simulink model "rtwdemo_cppencap"  (Simulink 7.6)
settings: Solver=FixedStepDiscrete  SolverMode=SingleTasking  StartTime=0.0  StopTime=100.0  FixedStep=0.1  RelTol=1e-3
PostLoadFcn:
  | rtwdemo_cppencap_data
libraries: rtwdemowidgets x1
Description:
  | C++ Classes for Models
settings Model: Creator=The MathWorks Inc.  CovMetricSettings=d  ExtModeAutoUpdateStatusClock=off
settings DataIOCC: SaveOutput=off  SaveTime=off  SignalLoggingName=sigsOut
settings OptimizationCC: InlineParams=on  InlineInvariantSignals=on  PassReuseOutputArgsAs=Individual arguments  StateBitsets=on  DataBitsets=on  UseTempVars=on  ZeroExternalMemoryAtStartup=off  ZeroInternalMemoryAtStartup=off  NoFixptDivByZeroProtection=on  EfficientFloat2IntCast=on  OptimizeModelRefInitCode=on  LifeSpan=1
settings DebuggingCC: SignalInfNanChecking=error  AlgebraicLoopMsg=error  ArtificialAlgebraicLoopMsg=error  UnderspecifiedInitializationDetection=Simplified  MergeDetectMultiDrivingBlocksExec=error  CheckExecutionContextPreStartOutputMsg=on  CheckExecutionContextRuntimeOutputMsg=on  BlockPriorityViolationMsg=error  MinStepSizeMsg=error  SolverPrmCheckMsg=error  InheritedTsInSrcMsg=error  DiscreteInheritContinuousMsg=error  SingleTaskRateTransMsg=error  TasksWithSamePriorityMsg=error  SigSpecEnsureSampleTimeMsg=error  CheckMatrixSingularityMsg=error  IntegerOverflowMsg=error  ParameterUnderflowMsg=error  ParameterPrecisionLossMsg=error  ParameterTunabilityLossMsg=error  UnderSpecifiedDataTypeMsg=error  UniqueDataStoreMsg=error  UnknownTsInhSupMsg=error  StrictBusMsg=ErrorOnBusTreatedAsVector
settings HardwareCC: ProdIntDivRoundTo=Zero  ProdEndianess=LittleEndian  ProdHWDeviceType=Generic->32-bit Embedded Processor  TargetHWDeviceType=Generic->32-bit Embedded Processor
settings SFSimCC: SimParseCustomCode=off
settings RTWCC: SystemTargetFile=ert.tlc  TLCOptions=-p0  TemplateMakefile=ert_default_tmf  Description=Real-Time Workshop Embedded Coder (no auto configuration)  GenerateReport=on  RTWVerbose=off  ProcessScript=ert_make_rtw_hook  IncludeHyperlinkInReport=on  LaunchReport=on  TargetLang=C++ (Encapsulated)  GenerateTraceInfo=on  GenerateTraceReport=on  GenerateTraceReportSl=on  GenerateTraceReportSf=on  GenerateTraceReportEml=on
settings CodeAppCC: ForceParamTrailComments=on  IgnoreTestpoints=on  MaxIdLength=128  SimulinkDataObjDesc=on  CustomSymbolStrGlobalVar=rt$N$M  CustomSymbolStrType=$N$M  CustomSymbolStrFcn=$N$M$F  CustomSymbolStrMacro=$N$M  InsertBlockDesc=on
settings ERTTargetCC: MultiwordLength=2048  GenerateSampleERTMain=on  IncludeMdlTerminateFcn=off  MultiInstanceERTCode=on  SupportNonFinite=off  SupportComplex=off  InlinedParameterPlacement=NonHierarchical  RootIOFormat=Structure reference  ERTCustomFileTemplate=example_file_process.tlc  ConvertIfToSwitch=off
settings ERTCPPComponent: GenerateDestructor=on  GenerateExternalIOAccessMethods=None  ParameterMemberVisibility=private  InternalMemberVisibility=private  GenerateParameterAccessMethods=None  GenerateInternalMemberAccessMethods=None  UseOperatorNewForModelRefRegistration=off

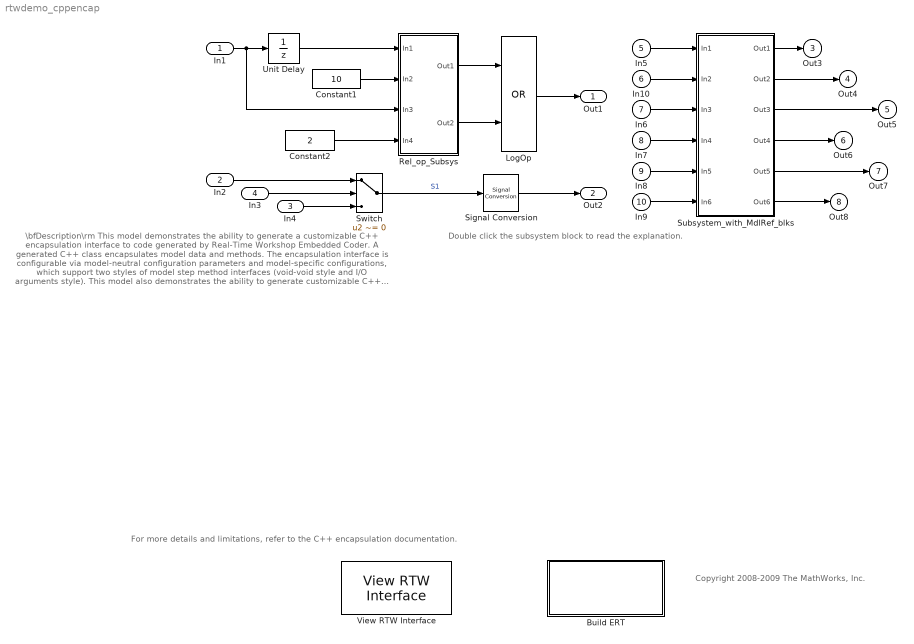
== system rtwdemo_cppencap ==
  note: \bfDescription\rm
      | This model demonstrates the ability to generate a customizable C++ encapsulation interface to code generated by
      | Real-Time Workshop Embedded Coder. A generated C++ class encapsulates model data and methods. The encapsulation
      | interface is configurable via model-neutral configuration parameters and model-specific configurations, which support two
      | styles of model step method interfaces (void-void style and I/O arguments style). This model also demonstrates the ability
      | to generate customizable C++ encapsulation interfaces for referenced models and for models to interact via those interfaces.
      | \bfInstructions\rm
      | 1. The model is preconfigured with a C++ encapsulation interface that defines root-level model input and output to be
      |     arguments on the step method, using the I/O arguments style interface. Generate code by double-clicking the blue
      |     button below.  An HTML report is displayed automatically.
      | 2. Inspect the source in the generated files using the hyperlinks embedded in the report. Also follow the hyperlinks for the
      |     code generated for the referenced models.
      | 3. To view or change the interface configuration, double-click the yellow button below. On the Code interface subpanel,
      |     select or clear the check boxes to change model-neutral settings, or click "Configure C++ Encapsulation Interface" to
      |     launch the model-specific configuration dialog box.
      |
      | To configure a new or existing model for C++ encapsulation, choose "ert.tlc" as the system target file on the Real-Time
      | Workshop page, and then set the Language to "C++ (Encapsulated)". Go to the Interface page to configure the C++
      | encapsulation interface for the model.
  note: Copyright 2008-2009 The MathWorks, Inc.
  note: For more details and limitations, refer to the C++ encapsulation documentation.
  note: Double click the subsystem block to read the explanation.
  In1 : Inport  OutDataTypeStr=double  PortDimensions=1  SampleTime=1
  In2 : Inport  Port=2  OutDataTypeStr=Bus: BusObject  BusOutputAsStruct=on
  In4 : Inport  Port=3  OutDataTypeStr=Bus: BusObject  BusOutputAsStruct=on
  In3 : Inport  Port=4  OutDataTypeStr=uint8  PortDimensions=1  SampleTime=1
  In5 : Inport  Port=5  OutDataTypeStr=double  PortDimensions=1  SampleTime=0.1
  In10 : Inport  Port=6  OutDataTypeStr=double  PortDimensions=1  SampleTime=0.1
  In6 : Inport  Port=7  OutDataTypeStr=double  PortDimensions=1  SampleTime=0.1
  In7 : Inport  Port=8  OutDataTypeStr=double  PortDimensions=1  SampleTime=0.1
  In8 : Inport  Port=9  OutDataTypeStr=double  PortDimensions=1  SampleTime=0.1
  In9 : Inport  Port=10  OutDataTypeStr=double  PortDimensions=1  SampleTime=0.1
  Build ERT : Subsystem  mask{attrib_overrides={}}
      mask prompts: attrib_overrides "List of attributes to preserve (cell of strings):"
      mask help: Enter the attributes of the configuration set that you want preserved. Otherwise, the default configuration script will override your current settings.
      settings: OpenFcn=|
      | if ~exist('rtwdemo_ert_cppencap', 'dir')
      |     disp('Creating working directory rtwdemo_ert_cppencap')
      |     mkdir('rtwdemo_ert_cppencap')
      | end
      | cd('rtwdemo_ert_cppencap');
      | 
      | overrides=get_param(gcb,'attrib_overrides');
      | refModelC='rtwdemo_cppencap_refc';
      | load_system(refModelC);
      | ori_cs_refc = getActiveConfigSet(refModelC);
      | tmp_cs_refc = ori_cs_refc.copy;
      | tmp_cs_refc.Name = 'tempcs4refc';
      | attachConfigSet(refModelC, tmp_cs_refc);
      | setActiveConfigSet(refModelC, 'tempcs4refc');
      | rtwconfiguredemo(refModelC,'noop',false,overrides);
      | 
      | setProp(tmp_cs_refc,'CustomSymbolStr','$R$N$M');
      | set_param(refModelC,'dirty','off');
      | 
      | refModelMiddle='rtwdemo_cppencap_refmid';
      | load_system(refModelMiddle);
      | ori_cs_refmid = getActiveConfigSet(refModelMiddle);
      | tmp_cs_refmid = ori_cs_refmid.copy;
      | tmp_cs_refmid.Name = 'tempcs4refmid';
      | attachConfigSet(refModelMiddle, tmp_cs_refmid);
      | setActiveConfigSet(refModelMiddle, 'tempcs4refmid');
      | rtwconfiguredemo(refModelMiddle,'noop',false,overrides);
      |  setProp(tmp_cs_refmid,'CustomSymbolStr','$R$N$M');
      | set_param(refModelMiddle,'dirty','off');
      | refModelBot='rtwdemo_cppencap_refbot';
      | load_system(refModelBot);
      | ori_cs_refbot = getActiveConfigSet(refModelBot);
      | tmp_cs_refbot = ori_cs_refbot.copy;
      | tmp_cs_refbot.Name = 'tempcs4refbot';
      | attachConfigSet(refModelBot, tmp_cs_refbot);
      | setActiveConfigSet(refModelBot, 'tempcs4refbot');
      | rtwconfiguredemo(refModelBot,'noop',false,overrides);
      | setProp(tmp_cs_refbot,'CustomSymbolStr','$R$N$M');
      | 
      | set_param(refModelBot,'dirty','off');
      | 
      | 
      | modeltop='rtwdemo_cppencap';
      | ori_cs_top=getActiveConfigSet(modeltop);
      | tmp_cs_top = ori_cs_top.copy;
      | tmp_cs_top.Name = 'tempcs4top';
      | attachConfigSet(modeltop, tmp_cs_top);
      | setActiveConfigSet(modeltop, 'tempcs4top');
      | 
      | rtwconfiguredemo(modeltop,'noop',false,overrides);
      | rtwbuilddemomodel(modeltop);
      | cd('..')
      | 
      | setActiveConfigSet(refModelC, ori_cs_refc.Name);     setActiveConfigSet(refModelMiddle, ori_cs_refmid.Name);
      | setActiveConfigSet(refModelBot, ori_cs_refbot.Name);
      | setActiveConfigSet(modeltop, ori_cs_top.Name);
      | tmp_cs_refc = detachConfigSet(refModelC, tmp_cs_refc.Name);
      | tmp_cs_refmid = detachConfigSet(refModelMiddle, tmp_cs_refmid.Name);
      | tmp_cs_refbot = detachConfigSet(refModelBot, tmp_cs_refbot.Name);
      | tmp_cs_top = detachConfigSet(modeltop, tmp_cs_top.Name);
      | 
      | set_param(modeltop,'dirty','off');
      | set_param(refModelC,'dirty','off');                               set_param(refModelMiddle,'dirty','off');
      | set_param(refModelBot,'dirty','off');
      | 
      | close_system(refModelC);
      | close_system(refModelMiddle);
      | close_system(refModelBot);
      | 
      | clear modeltop refModelC refModelMiddle refModelBot overrides ori_cs_refc ori_cs_refmid  ori_cs_refbot ori_cs_top tmp_cs_refc  tmp_cs_refmid tmp_cs_refbot tmp_cs_top;
      mask Display:
      | disp(['Generate Code Using\n',...
      | 	  'Real-Time Workshop\n',...
      | 	  'Embedded Coder\n'...
      | 	  '(double-click)'])
  Constant1 : Constant  Value=10  OutDataTypeStr=Inherit: Inherit via back propagation
  Constant2 : Constant  Value=2  OutDataTypeStr=Inherit: Inherit via back propagation
  LogOp : Logic  Operator=OR
  Rel_op_Subsys : Subsystem  TreatAsAtomicUnit=on
  Signal Conversion : SignalConversion  ConversionOutput=Virtual bus
  Subsystem_with_MdlRef_blks : Subsystem  TreatAsAtomicUnit=on
  Switch : Switch  Criteria=u2 ~= 0  ZeroCross=off
  Unit Delay : UnitDelay  X0=10  SampleTime=-1
  View RTW Interface : rtwdemowidgets/View RTW Interface  SystemSampleTime=-1
  Out1 : Outport
  Out2 : Outport  Port=2  OutDataTypeStr=Bus: BusObject
  Out3 : Outport  Port=3
  Out4 : Outport  Port=4
  Out5 : Outport  Port=5
  Out6 : Outport  Port=6
  Out7 : Outport  Port=7
  Out8 : Outport  Port=8
  wires:
  Constant2/1 -> Rel_op_Subsys/4(In4)
  In1/1 -> Rel_op_Subsys/3(In3), Unit Delay/1
  LogOp/1 -> Out1/1
  In2/1 -> Switch/1
  Switch/1 -> Signal Conversion/1  "S1"
  Signal Conversion/1 -> Out2/1
  In4/1 -> Switch/3
  In3/1 -> Switch/2
  Unit Delay/1 -> Rel_op_Subsys/1(In1)
  Constant1/1 -> Rel_op_Subsys/2(In2)
  Rel_op_Subsys/2(Out2) -> LogOp/2
  Rel_op_Subsys/1(Out1) -> LogOp/1
  Subsystem_with_MdlRef_blks/1(Out1) -> Out3/1
  In5/1 -> Subsystem_with_MdlRef_blks/1(In1)
  Subsystem_with_MdlRef_blks/2(Out2) -> Out4/1
  Subsystem_with_MdlRef_blks/3(Out3) -> Out5/1
  In6/1 -> Subsystem_with_MdlRef_blks/3(In3)
  Subsystem_with_MdlRef_blks/4(Out4) -> Out6/1
  In7/1 -> Subsystem_with_MdlRef_blks/4(In4)
  Subsystem_with_MdlRef_blks/5(Out5) -> Out7/1
  In8/1 -> Subsystem_with_MdlRef_blks/5(In5)
  Subsystem_with_MdlRef_blks/6(Out6) -> Out8/1
  In9/1 -> Subsystem_with_MdlRef_blks/6(In6)
  In10/1 -> Subsystem_with_MdlRef_blks/2(In2)

== system rtwdemo_cppencap/Build ERT ==

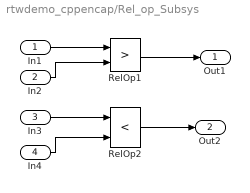
== system rtwdemo_cppencap/Rel_op_Subsys ==
  In1 : Inport
  In2 : Inport  Port=2
  In3 : Inport  Port=3
  In4 : Inport  Port=4
  RelOp1 : RelationalOperator  Operator=>  InputSameDT=on
  RelOp2 : RelationalOperator  Operator=<  InputSameDT=on
  Out1 : Outport
  Out2 : Outport  Port=2
  wires:
  In3/1 -> RelOp2/1
  In1/1 -> RelOp1/1
  RelOp1/1 -> Out1/1
  In2/1 -> RelOp1/2
  RelOp2/1 -> Out2/1
  In4/1 -> RelOp2/2

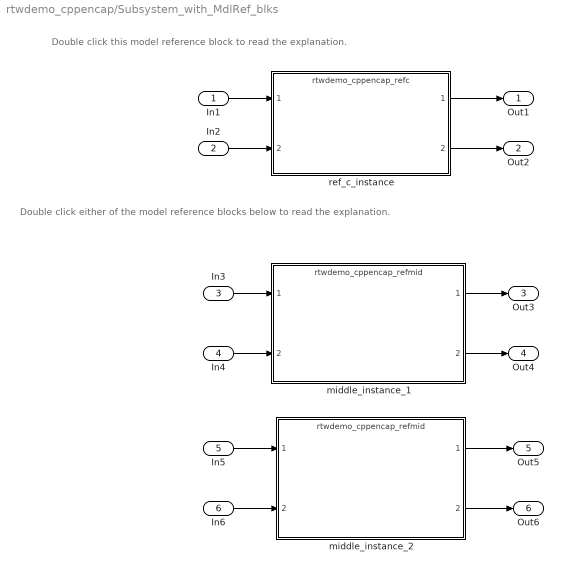
== system rtwdemo_cppencap/Subsystem_with_MdlRef_blks ==
  note: Double click this model reference block to read the explanation.
  note: Double click either of the model reference blocks below to read the
      | explanation.
  In1 : Inport  SampleTime=0.1
  In2 : Inport  Port=2
  In3 : Inport  Port=3
  In4 : Inport  Port=4
  In5 : Inport  Port=5
  In6 : Inport  Port=6
  middle_instance_1 : ModelReference  ModelNameDialog=rtwdemo_cppencap_refmid  SimulationMode=Accelerator  ModelReferenceVersion=1.323  CopyOfModelName=rtwdemo_cppencap_refmid
  middle_instance_2 : ModelReference  ModelNameDialog=rtwdemo_cppencap_refmid  SimulationMode=Accelerator  ModelReferenceVersion=1.323  CopyOfModelName=rtwdemo_cppencap_refmid
  ref_c_instance : ModelReference  ModelNameDialog=rtwdemo_cppencap_refc  SimulationMode=Accelerator  ModelReferenceVersion=1.310  CopyOfModelName=rtwdemo_cppencap_refc
  Out1 : Outport
  Out2 : Outport  Port=2
  Out3 : Outport  Port=3
  Out4 : Outport  Port=4
  Out5 : Outport  Port=5
  Out6 : Outport  Port=6
  wires:
  middle_instance_2/2 -> Out6/1
  In6/1 -> middle_instance_2/2
  middle_instance_2/1 -> Out5/1
  In5/1 -> middle_instance_2/1
  middle_instance_1/2 -> Out4/1
  In4/1 -> middle_instance_1/2
  middle_instance_1/1 -> Out3/1
  In3/1 -> middle_instance_1/1
  ref_c_instance/2 -> Out2/1
  In1/1 -> ref_c_instance/1
  ref_c_instance/1 -> Out1/1
  In2/1 -> ref_c_instance/2
